simulink model "Project3_Trial"  (R2021b)
settings: Solver=VariableStepAuto  StartTime=0.0  StopTime=Sim_Time  MaxStep=0.01  RelTol=1e-3
values from neighbouring files (symbols this model uses):
  b = 10    [Project3_Run_Trial.m]
  F = 1    [Project3_Run_Trial.m]
  k = 20    [Project3_Run_Trial.m]
  M = 1    [Project3_Run_Trial.m]
settings Model: Creator=rohitkharat  LastModifiedBy=rohitkharat

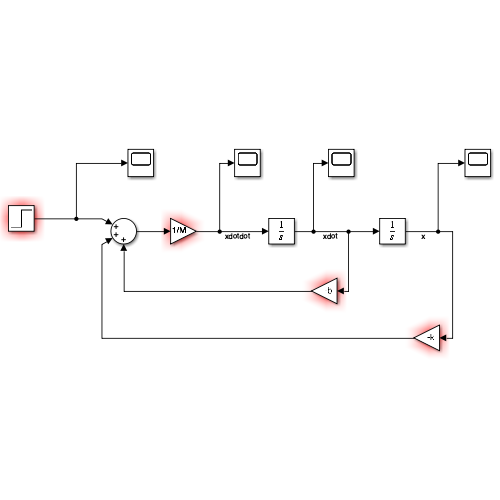
[thumbnail: Simulink's stored preview of the top-level diagram]
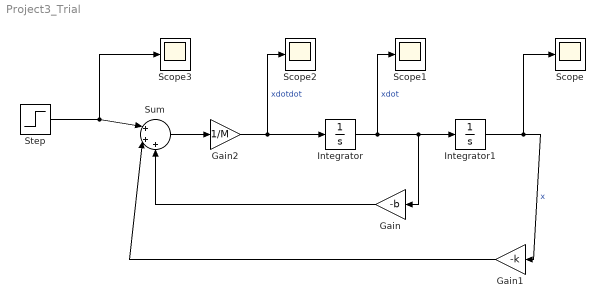
== system Project3_Trial ==
  Gain : Gain  Gain=-b
  Gain1 : Gain  Gain=-k
  Gain2 : Gain  Gain=1/M
  Integrator : Integrator
  Integrator1 : Integrator
  Scope{,1..3} (4 alike) : Scope
  Step : Step  After=F  SampleTime=0
  Sum : Sum  Inputs=|+++
  wires:
  Sum/1 -> Gain2/1
  Integrator/1 -> Scope1/1, Integrator1/1, Gain/1  "xdot"
  Integrator1/1 -> Scope/1, Gain1/1  "x"
  Step/1 -> Scope3/1, Sum/1
  Gain1/1 -> Sum/2
  Gain/1 -> Sum/3
  Gain2/1 -> Scope2/1, Integrator/1  "xdotdot"
